simulink model "bh_CONCEPT_rate_filter"  (R2016a)
settings: Solver=ode23s  StartTime=0.0  StopTime=10  FixedStep=0.001  RelTol=1e-5
libraries: dsparch4 x2, simulink x1
settings Model: Creator=bhorton  LastModifiedBy=bhorton
settings DataIOCC: SaveOutput=off  SignalLogging=off  DSMLogging=off  VisualizeSimOutput=off  SaveTime=off
settings DebuggingCC: AlgebraicLoopMsg=error  AllowSymbolicDim=off
settings ModelReferenceCC: PropagateSignalLabelsOutOfModel=off
settings GRTTargetCC: GeneratePreprocessorConditionals=Use local settings

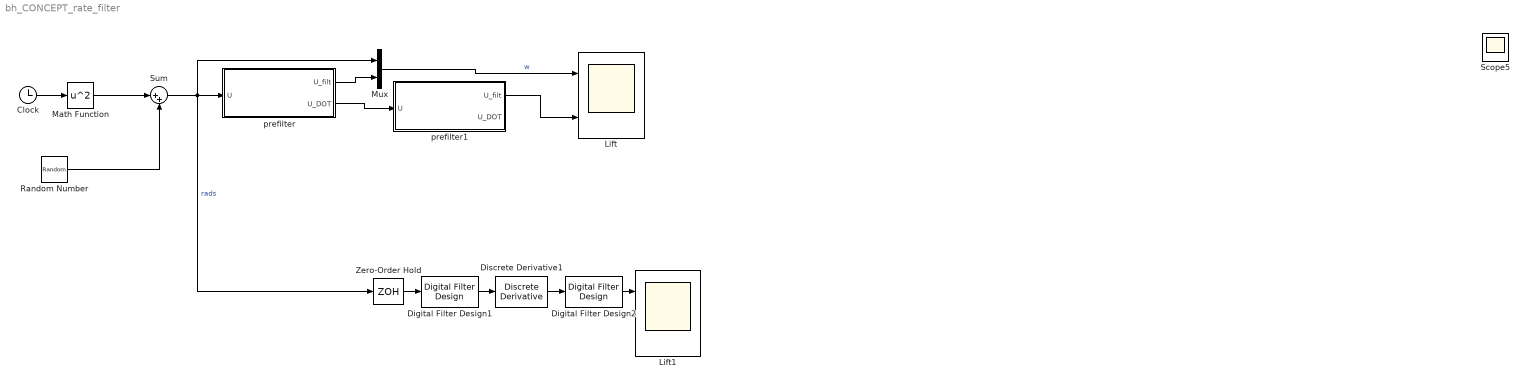
== system bh_CONCEPT_rate_filter ==
  Clock : Clock
  Digital Filter Design1 : dsparch4/Digital Filter Design  mwdsp_browser_bugfix_var=off
  Digital Filter Design2 : dsparch4/Digital Filter Design  mwdsp_browser_bugfix_var=off
  Discrete Derivative1 : simulink/Discrete/Discrete Derivative  gainval=1.0  ICPrevScaledInput=0.0  InputProcessing=Inherited  OutMin=[]  OutMax=[]  OutDataType=fixdt(1, 16)  OutScaling=2^-10  DoSatur=off
  Lift : Scope  NumInputPorts=2
  Lift1 : Scope  NumInputPorts=2
  Math Function : Math  Operator=square  SaturateOnIntegerOverflow=on
  Mux : Mux  Inputs=2
  Random Number : RandomNumber  SampleTime=0.01
  Sum : Sum  Inputs=|++
  Zero-Order Hold : ZeroOrderHold  SampleTime=1/100
  prefilter : Subsystem  mask(Derivative Estimation){wn=2*pi*2, p=1, dt=0}
      mask prompts: wn "Natural frequency, wn (rad/sec)"; p "Damping ratio, p"; dt "Sample time, dt (secs)"
      mask help:
      | A simple derivative estimator using a 2nd order representation between input and output.
      |
      | The integrators use a discrete FORWARd Euler rule, and a sample time needs to be specified.
      mask init:
      | str1 = sprintf('wn = %.2f', wn);
      | str2 = sprintf('p  = %.2f', p);
      | str3 = sprintf('dt = %.2f', dt);
      | str = char(str1,str2,str3);
      mask Display: disp(str)
  prefilter1 : Subsystem  mask(Derivative Estimation){wn=2*pi*2, p=1, dt=0}
      mask prompts: wn "Natural frequency, wn (rad/sec)"; p "Damping ratio, p"; dt "Sample time, dt (secs)"
      mask help:
      | A simple derivative estimator using a 2nd order representation between input and output.
      |
      | The integrators use a discrete FORWARd Euler rule, and a sample time needs to be specified.
      mask init:
      | str1 = sprintf('wn = %.2f', wn);
      | str2 = sprintf('p  = %.2f', p);
      | str3 = sprintf('dt = %.2f', dt);
      | str = char(str1,str2,str3);
      mask Display: disp(str)
  Scope5 : Scope
  wires:
  prefilter/1(U_filt) -> Mux/2
  Mux/1 -> Lift/1  "w"
  Clock/1 -> Math Function/1
  Math Function/1 -> Sum/1
  Random Number/1 -> Sum/2
  Sum/1 -> Zero-Order Hold/1, Mux/1, prefilter/1(U)  "rads"
  Digital Filter Design1/1 -> Discrete Derivative1/1
  Zero-Order Hold/1 -> Digital Filter Design1/1
  Discrete Derivative1/1 -> Digital Filter Design2/1
  Digital Filter Design2/1 -> Lift1/1
  prefilter/2(U_DOT) -> prefilter1/1(U)
  prefilter1/1(U_filt) -> Lift/2

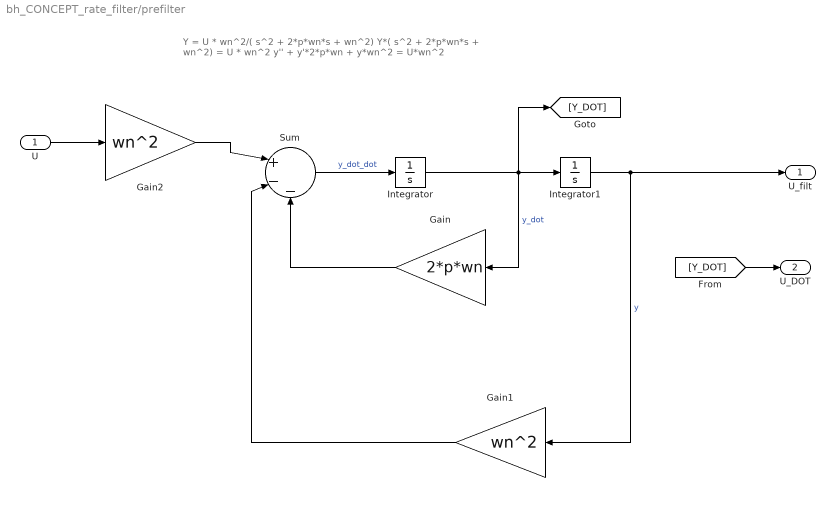
== system bh_CONCEPT_rate_filter/prefilter ==
  note: Y = U *     wn^2/( s^2 + 2*p*wn*s + wn^2)
      | Y*( s^2 + 2*p*wn*s + wn^2) = U * wn^2
      |
      | y'' + y'*2*p*wn + y*wn^2 = U*wn^2
  U : Inport
  Gain : Gain  Gain=2*p*wn
  Gain1 : Gain  Gain=wn^2
  Gain2 : Gain  Gain=wn^2
  Integrator : Integrator
  Integrator1 : Integrator
  Sum : Sum  Inputs=|+--
  U_filt : Outport
  U_DOT : Outport  Port=2
  wires:
  Integrator/1 -> Integrator1/1, [Y_DOT], Gain/1  "y_dot"
  Sum/1 -> Integrator/1  "y_dot_dot"
  Integrator1/1 -> Gain1/1, U_filt/1  "y"
  U/1 -> Gain2/1
  Gain2/1 -> Sum/1
  Gain/1 -> Sum/3
  Gain1/1 -> Sum/2
  [Y_DOT] -> U_DOT/1

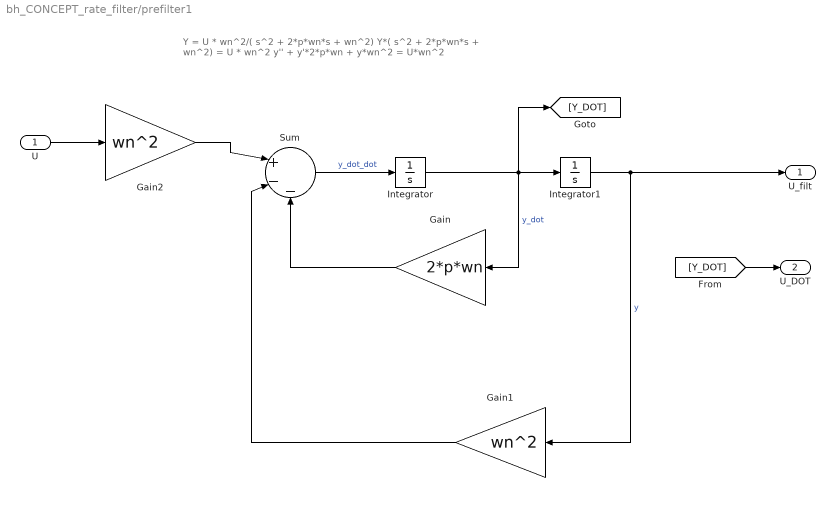
== system bh_CONCEPT_rate_filter/prefilter1 ==
  note: Y = U *     wn^2/( s^2 + 2*p*wn*s + wn^2)
      | Y*( s^2 + 2*p*wn*s + wn^2) = U * wn^2
      |
      | y'' + y'*2*p*wn + y*wn^2 = U*wn^2
  U : Inport
  Gain : Gain  Gain=2*p*wn
  Gain1 : Gain  Gain=wn^2
  Gain2 : Gain  Gain=wn^2
  Integrator : Integrator
  Integrator1 : Integrator
  Sum : Sum  Inputs=|+--
  U_filt : Outport
  U_DOT : Outport  Port=2
  wires:
  Integrator/1 -> Integrator1/1, [Y_DOT], Gain/1  "y_dot"
  Sum/1 -> Integrator/1  "y_dot_dot"
  Integrator1/1 -> Gain1/1, U_filt/1  "y"
  U/1 -> Gain2/1
  Gain2/1 -> Sum/1
  Gain/1 -> Sum/3
  Gain1/1 -> Sum/2
  [Y_DOT] -> U_DOT/1
